simulink subsystem "canard_forces_torques"  (R2026a)
settings: Solver=VariableStepAuto
undefined symbols (not defined in the file or in its folder): canard_area, canard_CL_alpha_data, canard_CL_alpha_input, canard_CL_data, canard_CL_Mach_input, canard_pos_r_mean, canard_pos_x, canard_roll_reversal_time, roll_rev_grid_active
settings Model: Creator=trist  LastModifiedBy=trist

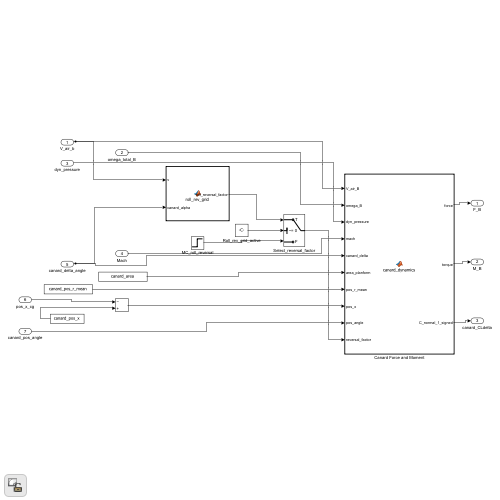
[thumbnail: Simulink's stored preview of the top-level diagram]
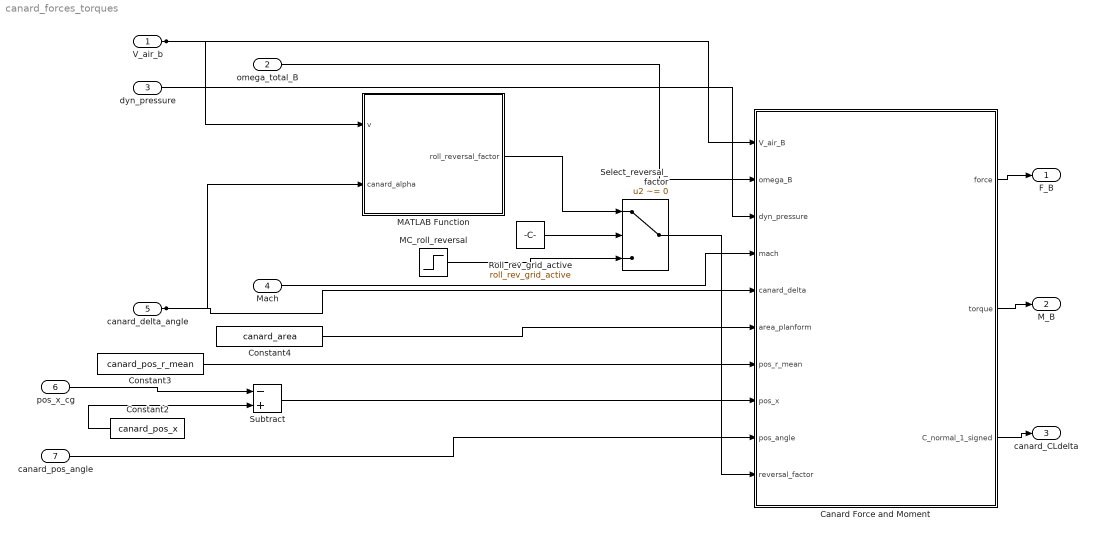
== system canard_forces_torques ==
  V_air_b : Inport
  omega_total_B : Inport  Port=2
  "dyn_pressure " : Inport  Port=3
  "Mach " : Inport  Port=4
  canard_delta_angle : Inport  Port=5
  pos_x_cg : Inport  Port=6
  canard_pos_angle : Inport  Port=7
  Canard Force and Moment : MATLAB Function  TreatAsAtomicUnit=on
  Constant2 : Constant  Value=canard_pos_x
  Constant3 : Constant  Value=canard_pos_r_mean
  Constant4 : Constant  Value=canard_area
  MATLAB Function : MATLAB Function  TreatAsAtomicUnit=on
  MC_roll_reversal : Step  Time=canard_roll_reversal_time  InitialValue=1  FinalValue=canard_roll_reversal_factor  SampleTime=0
  Roll_rev_grid_active : Constant  Value=roll_rev_grid_active
  Select_reversal_factor : Switch  Criteria=u2 ~= 0
  Subtract : Sum  Inputs=-+
  F_B : Outport  VectorParamsAs1DForOutWhenUnconnected=off
  M_B : Outport  Port=2  VectorParamsAs1DForOutWhenUnconnected=off
  canard_CLdelta : Outport  Port=3  VectorParamsAs1DForOutWhenUnconnected=off
  wires:
  Select_reversal_factor/1 -> Canard Force and Moment/10(reversal_factor)
  MC_roll_reversal/1 -> Select_reversal_factor/3
  Roll_rev_grid_active/1 -> Select_reversal_factor/2
  Constant4/1 -> Canard Force and Moment/6(area_planform)
  Constant3/1 -> Canard Force and Moment/7(pos_r_mean)
  Canard Force and Moment/1(force) -> F_B/1
  MATLAB Function/1(roll_reversal_factor) -> Select_reversal_factor/1
  Subtract/1 -> Canard Force and Moment/8(pos_x)
  pos_x_cg/1 -> Subtract/1
  Constant2/1 -> Subtract/2
  canard_pos_angle/1 -> Canard Force and Moment/9(pos_angle)
  omega_total_B/1 -> Canard Force and Moment/2(omega_B)
  Canard Force and Moment/3(C_normal_1_signed) -> canard_CLdelta/1
  "dyn_pressure "/1 -> Canard Force and Moment/3(dyn_pressure)
  "Mach "/1 -> Canard Force and Moment/4(mach)
  canard_delta_angle/1 -> MATLAB Function/2(canard_alpha), Canard Force and Moment/5(canard_delta)
  V_air_b/1 -> MATLAB Function/1(v), Canard Force and Moment/1(V_air_B)
  Canard Force and Moment/2(torque) -> M_B/1

== matlab function canard_forces_torques/Canard Force and Moment ==
  data: force output; V_air_B input; omega_B input; dyn_pressure input; mach input; canard_delta input; area_planform input; pos_r_mean input; pos_x input; pos_angle input; torque output; C_normal_1_signed output; reversal_factor input; canard_CL_Mach_input parameter size=[1 201]; canard_CL_alpha_input parameter size=[1 151]; canard_CL_data parameter size=[151 201]; canard_CL_alpha_data parameter size=[151 201]
function [force, torque, C_normal_1_signed] = canard_dynamics(V_air_B, omega_B, dyn_pressure, mach, canard_delta, area_planform, pos_r_mean, pos_x, pos_angle, reversal_factor, canard_CL_Mach_input, canard_CL_alpha_input, canard_CL_data, canard_CL_alpha_data)
    % canard position
    pos = [pos_x; pos_r_mean*cos(deg2rad(pos_angle)); pos_r_mean*sin(deg2rad(pos_angle))];

    % relative velocity
    Vrel = V_air_B + cross(omega_B, pos);
    
    % local incidence 
    alpha_local = atan(Vrel(3) / Vrel(1));
    incidence = canard_delta - alpha_local;

    [C_normal_1, CL_alpha] = aerosurface_canard_online(mach, incidence, canard_CL_Mach_input, canard_CL_alpha_input, canard_CL_data, canard_CL_alpha_data) ;
    C_normal_1_signed = CL_alpha * sign(Vrel(1) + 1e-1) * reversal_factor;
    force = C_normal_1 * sign(incidence) * sign(Vrel(1)) * area_planform * dyn_pressure * [0; 0; 1] * reversal_factor;

    torque = cross(pos, force);
end

== matlab function canard_forces_torques/MATLAB Function ==
  data: roll_reversal_factor output; v input; canard_alpha input; roll_rev_grid_active parameter
function roll_reversal_factor = roll_rev_grid(v, canard_alpha, roll_rev_grid_active)
    
    airspeed = norm(v);

    if roll_rev_grid_active == false
        roll_reversal_factor = 1;
        return;
    end
    
    roll_reversal_factor = rev_grid(airspeed, canard_alpha);

end
